simulink model "Assignment1"  (R2020a)
settings: Solver=FixedStepAuto  StartTime=0.0  StopTime=5  FixedStep=1e-3  RelTol=1e-3  EnableMultiTasking=on
model workspace (MAT data in the model file):
  ATR_CMP_REF_PWM_PERCENTAGE = 50
  PACING_REF_PWM_DUTY_PERCENTAGE = 50
  VENT_CMP_REF_PWM_PERCENTAGE = 50
undefined symbols (not defined in the file or in its folder): A0, A1, A2, A3, A4, D0, D1, PTB10, PTB11, PTB2, PTB3, PTC11, PTC16, PTC17
libraries: frdmk64flib x7
settings Model: ExtModeTrigDuration=5  OrderedModelArguments=off  Creator=John  LastModifiedBy=changhaibian
settings OptimizationCC: EnhancedBackFolding=on  PassReuseOutputArgsAs=Individual arguments  ZeroExternalMemoryAtStartup=off  ZeroInternalMemoryAtStartup=off  MaxStackSize=64  OptimizeBlockOrder=speed  DifferentSizesBufferReuse=on  OptimizationCustomize=off  EfficientTunableParamExpr=on
settings DebuggingCC: ParameterTunabilityLossMsg=error
settings HardwareCC: ProdBitPerPointer=32  ProdBitPerSizeT=32  ProdBitPerPtrDiffT=32  ProdLargestAtomicInteger=Long  ProdLargestAtomicFloat=Double  ProdWordSize=32  ProdHWDeviceType=ARM Compatible->ARM Cortex
settings SFSimCC: MATLABDynamicMemAlloc=off
settings RTWCC: SystemTargetFile=ert.tlc  HardwareBoard=NXP FRDM-K64F  TemplateMakefile=ert_default_tmf  Toolchain=GNU Tools for ARM Embedded Processors
settings CodeAppCC: ForceParamTrailComments=on  IgnoreCustomStorageClasses=off  OperatorAnnotations=on  SimulinkDataObjDesc=on  SFDataObjDesc=on  InsertBlockDesc=on

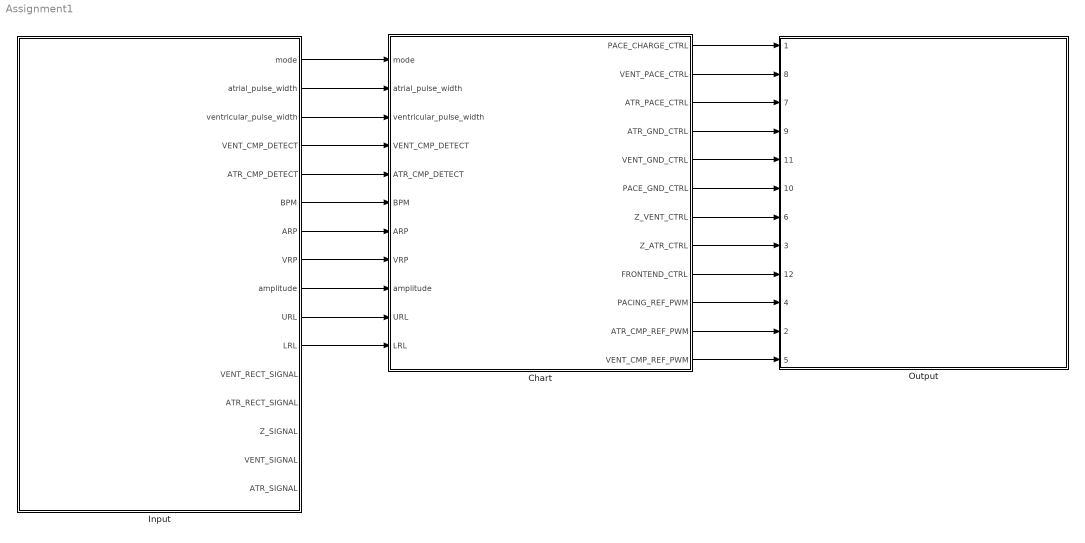
== system Assignment1 ==
  Chart : Stateflow chart  TreatAsAtomicUnit=on
  Input : Subsystem
  Output : Subsystem  ReferencedSubsystem=k64f_subsystem
      settings: PortSchema="{\"entries\":[{\"content\":{\"sides\":[{\"content\":{\"connectorIds\":[\"In1\",\"In8\",\"In7\",\"In9\",\"In11\",\"In10\",\"In6\",\"In3\",\"In12\",\"In4\",\"In2\",\"In5\"]},\"type\":\"ConnectorPlacement.EquallySpacedRectSide\",\"uuid\":\"5fe5e99a-062c-46b1-a2f7-269af42544f1\"},{\"content\":{\"connectorIds\":[],\"side\":\"RIGHT\"},\"type\":\"ConnectorPlacement.EquallySpacedRectSide\",\"uuid\":\"5e0ab6a5-47b7-4042-9674-b1d9edf072a6\"},{\"content\":{\"connectorIds\":[],\"side\":\"TOP\"},\"type\":\"ConnectorPlacement.EquallySpacedRectSide\",\"uuid\":\"d92f43c7-fab1-41f9-bb4e-b34a1c9b65d6\"}]},\"type\":\"ConnectorPlacement.EquallySpacedConnector\",\"uuid\":\"e370713e-2556-4eda-81ac-c10d9f2319e9\"}],\"packageUris\":[\"http://schema.mathworks.com/mf0/Connector/19700101\"],\"version\":\"1.0\"}"
  wires:
  Input/1(mode) -> Chart/1(mode)
  Chart/10(PACING_REF_PWM) -> Output/4
  Input/2(atrial_pulse_width) -> Chart/2(atrial_pulse_width)
  Input/3(ventricular_pulse_width) -> Chart/3(ventricular_pulse_width)
  Chart/8(Z_ATR_CTRL) -> Output/3
  Chart/7(Z_VENT_CTRL) -> Output/6
  Chart/4(ATR_GND_CTRL) -> Output/9
  Chart/3(ATR_PACE_CTRL) -> Output/7
  Chart/5(VENT_GND_CTRL) -> Output/11
  Chart/2(VENT_PACE_CTRL) -> Output/8
  Chart/1(PACE_CHARGE_CTRL) -> Output/1
  Chart/6(PACE_GND_CTRL) -> Output/10
  Chart/11(ATR_CMP_REF_PWM) -> Output/2
  Chart/12(VENT_CMP_REF_PWM) -> Output/5
  Chart/9(FRONTEND_CTRL) -> Output/12
  Input/6(BPM) -> Chart/6(BPM)
  Input/4(VENT_CMP_DETECT) -> Chart/4(VENT_CMP_DETECT)
  Input/5(ATR_CMP_DETECT) -> Chart/5(ATR_CMP_DETECT)
  Input/7(ARP) -> Chart/7(ARP)
  Input/8(VRP) -> Chart/8(VRP)
  Input/9(amplitude) -> Chart/9(amplitude)
  Input/10(URL) -> Chart/10(URL)
  Input/11(LRL) -> Chart/11(LRL)

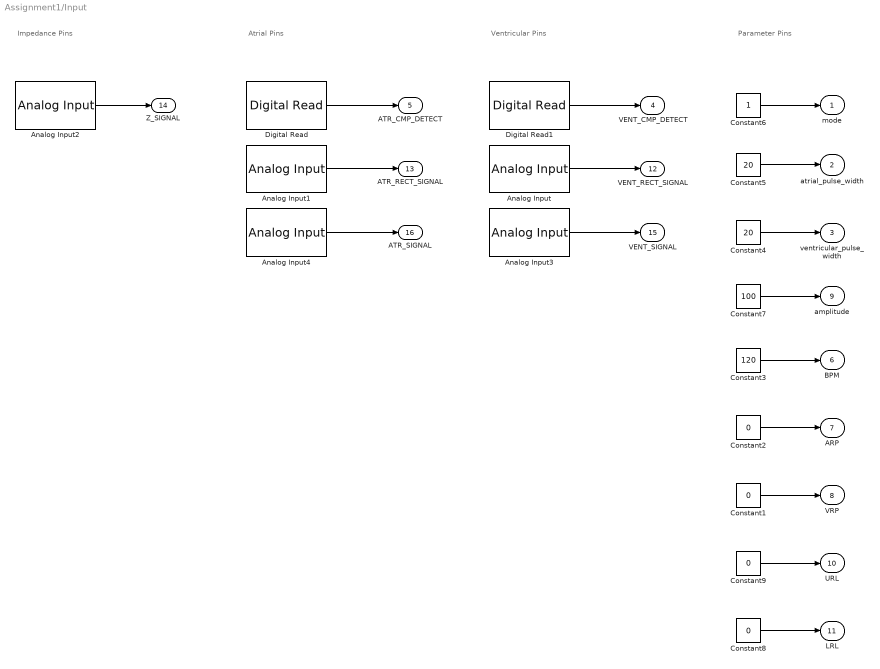
== system Assignment1/Input ==
  note: Ventricular Pins
  note: Atrial Pins
  note: Impedance Pins
  note: Parameter Pins
  Analog Input : frdmk64flib/Analog Input  Whichpin=PTC11 (A4)  SampleTime=-1
  Analog Input1 : frdmk64flib/Analog Input  Whichpin=PTB11 (A3)  SampleTime=-1
  Analog Input2 : frdmk64flib/Analog Input  Whichpin=PTB10 (A2)  SampleTime=-1
  Analog Input3 : frdmk64flib/Analog Input  Whichpin=PTB3 (A1)  SampleTime=-1
  Analog Input4 : frdmk64flib/Analog Input  Whichpin=PTB2 (A0)  SampleTime=-1
  Constant{1..2,8..9} (4 alike) : Constant  Value=0
  Constant3 : Constant  Value=120
  Constant4 : Constant  Value=20
  Constant5 : Constant  Value=20
  Constant6 : Constant
  Constant7 : Constant  Value=100
  Digital Read : frdmk64flib/Digital Read  Whichpin=PTC16 (D0)  SampleTime=-1
  Digital Read1 : frdmk64flib/Digital Read  Whichpin=PTC17 (D1)  SampleTime=-1
  mode : Outport
  atrial_pulse_width : Outport  Port=2
  ventricular_pulse_width : Outport  Port=3
  VENT_CMP_DETECT : Outport  Port=4
  ATR_CMP_DETECT : Outport  Port=5
  BPM : Outport  Port=6
  ARP : Outport  Port=7
  VRP : Outport  Port=8
  amplitude : Outport  Port=9
  URL : Outport  Port=10
  LRL : Outport  Port=11
  VENT_RECT_SIGNAL : Outport  Port=12
  ATR_RECT_SIGNAL : Outport  Port=13
  Z_SIGNAL : Outport  Port=14
  VENT_SIGNAL : Outport  Port=15
  ATR_SIGNAL : Outport  Port=16
  wires:
  Analog Input4/1 -> ATR_SIGNAL/1
  Analog Input2/1 -> Z_SIGNAL/1
  Analog Input3/1 -> VENT_SIGNAL/1
  Analog Input/1 -> VENT_RECT_SIGNAL/1
  Digital Read1/1 -> VENT_CMP_DETECT/1
  Digital Read/1 -> ATR_CMP_DETECT/1
  Analog Input1/1 -> ATR_RECT_SIGNAL/1
  Constant6/1 -> mode/1
  Constant5/1 -> atrial_pulse_width/1
  Constant4/1 -> ventricular_pulse_width/1
  Constant3/1 -> BPM/1
  Constant1/1 -> VRP/1
  Constant2/1 -> ARP/1
  Constant7/1 -> amplitude/1
  Constant9/1 -> URL/1
  Constant8/1 -> LRL/1

== stateflow chart Assignment1/Chart ==
  state AAI
    state delay
    state AOO_Charge
      entry:
      PACING_REF_PWM = amplitude;
      ATR_CMP_REF_PWM = 70;
      PACE_CHARGE_CTRL = 1;
      PACE_GND_CTRL = 1;
      ATR_PACE_CTRL = 0;
      ATR_GND_CTRL = 1;
      VENT_PACE_CTRL = 0;
      VENT_GND_CTRL = 0;
      Z_ATR_CTRL = 0;
      Z_VENT_CTRL =0;
      FRONTEND_CTRL = 0;
    state sense
      entry:
      FRONTEND_CTRL = 1;
    state Atrial_Pacing
      entry:
      PACING_REF_PWM = amplitude;
      ATR_CMP_REF_PWM = 70;
      PACE_CHARGE_CTRL = 0;
      PACE_GND_CTRL = 1;
      ATR_PACE_CTRL = 1;
      ATR_GND_CTRL = 0;
      VENT_PACE_CTRL = 0;
      VENT_GND_CTRL = 0;
      Z_ATR_CTRL = 0;
      Z_VENT_CTRL = 0;
    (default) -> AAI.AOO_Charge
    AAI.delay -> AAI.sense : [after(ARP,msec)]
    AAI.sense -> AAI.delay [order 1] : [ATR_CMP_DETECT == 1]
    AAI.AOO_Charge -> AAI.sense
    AAI.sense -> AAI.Atrial_Pacing [order 2] : [after((60000/BPM) - atrial_pulse_width + ARP,msec) && ATR_CMP_DETECT == 0]
    AAI.Atrial_Pacing -> AAI.AOO_Charge : [after(atrial_pulse_width,msec)]
  state VVI
    state delay
    state VVI_Charge
      entry:
      PACING_REF_PWM = amplitude;
      VENT_CMP_REF_PWM = 70;
      PACE_CHARGE_CTRL = 1;
      PACE_GND_CTRL = 1;
      ATR_PACE_CTRL = 0;
      ATR_GND_CTRL = 0;
      VENT_PACE_CTRL = 0;
      VENT_GND_CTRL = 1;
      Z_ATR_CTRL = 0;
      Z_VENT_CTRL =0;
    state sense
      entry:
      FRONTEND_CTRL = 1;
    state Ventricular_Pacing
      entry:
      PACING_REF_PWM = amplitude;
      VENT_CMP_REF_PWM = 70;
      PACE_CHARGE_CTRL = 0;
      PACE_GND_CTRL = 1;
      ATR_PACE_CTRL = 0;
      ATR_GND_CTRL = 0;
      Z_ATR_CTRL = 0;
      Z_VENT_CTRL = 0;
      VENT_PACE_CTRL = 1;
      VENT_GND_CTRL = 0;
    (default) -> VVI_Charge
    VVI.delay -> VVI.sense : [after(VRP,msec)]
    VVI.sense -> VVI.delay [order 1] : [VENT_CMP_DETECT == 1]
    VVI_Charge -> VVI.sense
    VVI.sense -> VVI.Ventricular_Pacing [order 2] : [after((60000/BPM) - ventricular_pulse_width + VRP + URL,msec) && VENT_CMP_DETECT == 0]
    VVI.Ventricular_Pacing -> VVI_Charge : [after(ventricular_pulse_width,msec)]
  state AOO
    state AOO_Charge
      entry:
      PACING_REF_PWM = amplitude;
      ATR_CMP_REF_PWM = 70;
      PACE_CHARGE_CTRL = 1;
      PACE_GND_CTRL = 1;
      ATR_PACE_CTRL = 0;
      ATR_GND_CTRL = 1;
      VENT_PACE_CTRL = 0;
      VENT_GND_CTRL = 0;
      Z_ATR_CTRL = 0;
      Z_VENT_CTRL =0;
      FRONTEND_CTRL = 0;
    state Atrial_Pacing
      entry:
      PACING_REF_PWM = amplitude;
      ATR_CMP_REF_PWM = 70;
      PACE_CHARGE_CTRL = 0;
      PACE_GND_CTRL = 1;
      ATR_PACE_CTRL = 1;
      ATR_GND_CTRL = 0;
      VENT_PACE_CTRL = 0;
      VENT_GND_CTRL = 0;
      Z_ATR_CTRL = 0;
      Z_VENT_CTRL = 0;
    (default) -> AOO.AOO_Charge
    AOO.AOO_Charge -> AOO.Atrial_Pacing : [after((60000/BPM) - atrial_pulse_width,msec)]
    AOO.Atrial_Pacing -> AOO.AOO_Charge : [after(atrial_pulse_width,msec)]
  state OFF
    entry:
    ATR_PACE_CTRL = 0;
    VENT_PACE_CTRL = 0;
  state VOO
    state VOO_Charge
      entry:
      PACING_REF_PWM = amplitude;
      VENT_CMP_REF_PWM = 70;
      PACE_CHARGE_CTRL = 1;
      PACE_GND_CTRL = 1;
      ATR_PACE_CTRL = 0;
      ATR_GND_CTRL = 0;
      VENT_PACE_CTRL = 0;
      VENT_GND_CTRL = 1;
      Z_ATR_CTRL = 0;
      Z_VENT_CTRL =0;
      FRONTEND_CTRL = 0;
    state Ventricular_Pacing
      entry:
      PACING_REF_PWM = amplitude;
      VENT_CMP_REF_PWM = 70;
      PACE_CHARGE_CTRL = 0;
      PACE_GND_CTRL = 1;
      ATR_PACE_CTRL = 0;
      ATR_GND_CTRL = 0;
      Z_ATR_CTRL = 0;
      Z_VENT_CTRL = 0;
      VENT_PACE_CTRL = 1;
      VENT_GND_CTRL = 0;
    (default) -> VOO_Charge
    VOO_Charge -> VOO.Ventricular_Pacing : [after((60000/BPM) - ventricular_pulse_width +LRL,msec)]
    VOO.Ventricular_Pacing -> VOO_Charge : [after(ventricular_pulse_width,msec)]
  AAI -> OFF : [mode ~= 3]
  OFF -> AAI [order 1] : [mode == 3]
  (default) -> OFF
  AOO -> OFF : [mode ~= 1]
  OFF -> VVI [order 3] : [mode == 4]
  OFF -> AOO [order 2] : [mode == 1]
  VVI -> OFF : [mode ~= 4]
  VOO -> OFF : [mode ~= 2]
  OFF -> VOO [order 4] : [mode == 2]
  data: PACE_CHARGE_CTRL output; VENT_PACE_CTRL output; ATR_PACE_CTRL output; ATR_GND_CTRL output; VENT_GND_CTRL output; PACE_GND_CTRL output; mode input; Z_VENT_CTRL output; Z_ATR_CTRL output; atrial_pulse_width input; ventricular_pulse_width input; VENT_CMP_DETECT input; ATR_CMP_DETECT input; FRONTEND_CTRL output; BPM input; PACING_REF_PWM output; ATR_CMP_REF_PWM output; VENT_CMP_REF_PWM output; ARP input; VRP input; amplitude input; URL input; LRL input
